simulink model "model"  (Simulink 7.4)
settings: Solver=ode45  StartTime=0.0  StopTime=15  MaxStep=2e-2  RelTol=1e-3
values from neighbouring files (symbols this model uses):
  Bm = 3e-6    (= 3e-06)    [beammodelparameters.m]    (also in project.mat)
  g = 9.8    [beammodelparameters.m]    (also in project.mat)
  Gv = 4    [beammodelparameters.m]    (also in project.mat)
  Jeff = Jm + Jg + Js    (= 5.66e-05)    [beammodelparameters.m]    (also in project.mat)
  K = (2/5)*(R/r)^2    (= 1.11111111111)    [beammodelparameters.m]    (also in project.mat)
  Ks = 10    [beammodelparameters.m]    (also in project.mat)
  Kt = 0.125    [beammodelparameters.m]    (also in project.mat = 0.225)
  Lm = 7.5e-3    (= 0.0075)    [beammodelparameters.m]    (also in project.mat = 0.025)
  M = 1 + (2/5)*(R/r)^2    (= 2.11111111111)    [beammodelparameters.m]    (also in lamdesign.m = p(nd+1:end).'; project.mat)
  N = 100    [beammodelparameters.m]    (also in lamdesign.m = [zeros(nd-nn,1);N]; project.mat)
  Rm = 4    [beammodelparameters.m]    (also in project.mat = 8)
  theta_o = 0.1    [beammodelparameters.m]    (also in project.mat)
  Vlim = 50    [beammodelparameters.m]    (also in project.mat)
  x_o = 0.25    [beammodelparameters.m]    (also in project.mat)
undefined symbols (not defined in the file or in its folder): Fn, Fp
settings Model: Creator=Duane  LastModifiedBy=Cam  ExtModeAutoUpdateStatusClock=off
settings DebuggingCC: SolverPrmCheckMsg=none

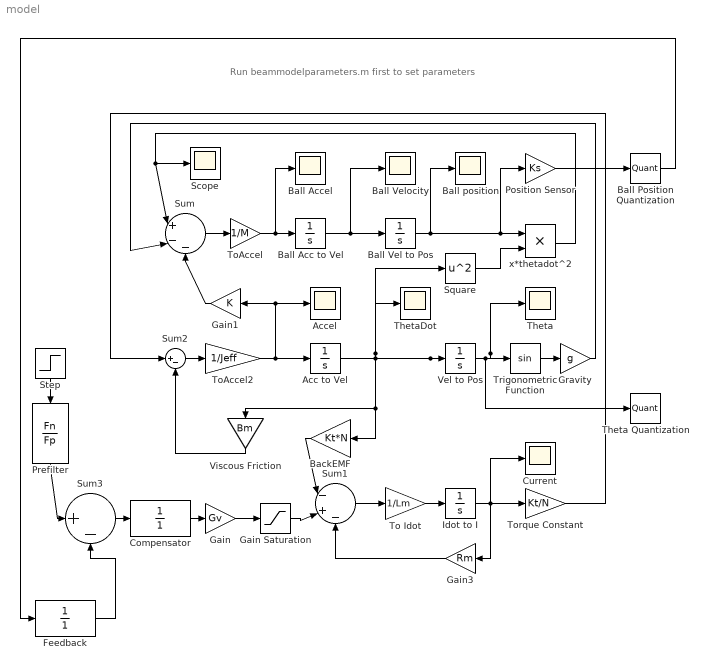
== system model ==
  note: Run beammodelparameters.m first to set parameters
  Acc to Vel : Integrator
  Accel : Scope
      settings: SaveName=ScopeData5
  BackEMF : Gain  Gain=Kt*N  ParameterDataType=fixdt(1, 16)  ParameterScaling=2^0  OutDataType=fixdt(1, 16)  OutScaling=2^0
  Ball Acc to Vel : Integrator
  Ball Accel : Scope
      settings: SaveName=ScopeData6
  Ball Position Quantization : Quantizer  QuantizationInterval=Xquant
  Ball Vel to Pos : Integrator  InitialCondition=x_o
  Ball Velocity : Scope
  Ball position : Scope
  Compensator : TransferFcn  Numerator=1  Denominator=1
  Current : Scope
      settings: SaveName=ScopeData4
  Feedback : TransferFcn  Numerator=1  Denominator=1
  Gain : Gain  Gain=Gv  ParameterDataType=fixdt(1, 16)  ParameterScaling=2^0  OutDataType=fixdt(1, 16)  OutScaling=2^0
  Gain Saturation : Saturate  UpperLimit=Vlim  LowerLimit=-Vlim  OutDataType=fixdt(1, 16)  OutScaling=2^0
  Gain1 : Gain  Gain=K  ParameterDataType=fixdt(1, 16)  ParameterScaling=2^0  OutDataType=fixdt(1, 16)  OutScaling=2^0
  Gain3 : Gain  Gain=Rm  ParameterDataType=fixdt(1, 16)  ParameterScaling=2^0  OutDataType=fixdt(1, 16)  OutScaling=2^0
  Gravity : Gain  Gain=g  ParameterDataType=fixdt(1, 16)  ParameterScaling=2^0  OutDataType=fixdt(1, 16)  OutScaling=2^0
  Idot to I : Integrator
  Position Sensor : Gain  Gain=Ks  ParameterDataType=fixdt(1, 16)  ParameterScaling=2^0  OutDataType=fixdt(1, 16)  OutScaling=2^0
  Prefilter : TransferFcn  Numerator=Fn  Denominator=Fp
  Scope : Scope
      settings: SaveName=ScopeData7
  Square : Math  Operator=square  OutDataType=fixdt(1, 16)  OutScaling=2^0  SaturateOnIntegerOverflow=on
  Step : Step  After=.05  SampleTime=0
  Sum : Sum  Inputs=|+--  OutDataType=fixdt(1, 16)  OutScaling=2^0
  Sum1 : Sum  Inputs=|-+-  OutDataType=fixdt(1, 16)  OutScaling=2^0
  Sum2 : Sum  Inputs=|+-  OutDataType=fixdt(1, 16)  OutScaling=2^0
  Sum3 : Sum  Inputs=|+-  OutDataType=fixdt(1, 16)  OutScaling=2^0
  Theta : Scope
      settings: SaveName=ScopeData2
  Theta Quantization : Quantizer  QuantizationInterval=Tquant
  ThetaDot : Scope
      settings: SaveName=ScopeData3
  To Idot : Gain  Gain=1/Lm  ParameterDataType=fixdt(1, 16)  ParameterScaling=2^0  OutDataType=fixdt(1, 16)  OutScaling=2^0
  ToAccel : Gain  Gain=1/M  ParameterDataType=fixdt(1, 16)  ParameterScaling=2^0  OutDataType=fixdt(1, 16)  OutScaling=2^0
  ToAccel2 : Gain  Gain=1/Jeff  ParameterDataType=fixdt(1, 16)  ParameterScaling=2^0  OutDataType=fixdt(1, 16)  OutScaling=2^0
  Torque Constant : Gain  Gain=Kt/N  ParameterDataType=fixdt(1, 16)  ParameterScaling=2^0  OutDataType=fixdt(1, 16)  OutScaling=2^0
  Trigonometric Function : Trigonometry
  Vel to Pos : Integrator  InitialCondition=theta_o
  Viscous Friction : Gain  Gain=Bm  ParameterDataType=fixdt(1, 16)  ParameterScaling=2^0  OutDataType=fixdt(1, 16)  OutScaling=2^0
  x*thetadot^2 : Product  Inputs=**  OutDataType=fixdt(1, 16)  OutScaling=2^-10
  wires:
  Ball Acc to Vel/1 -> Ball Vel to Pos/1, Ball Velocity/1
  Vel to Pos/1 -> Theta/1, Trigonometric Function/1, Theta Quantization/1
  ToAccel/1 -> Ball Acc to Vel/1, Ball Accel/1
  Sum/1 -> ToAccel/1
  Square/1 -> x*thetadot^2/2
  Ball Vel to Pos/1 -> Ball position/1, x*thetadot^2/1, Position Sensor/1
  x*thetadot^2/1 -> Sum/1, Scope/1
  Acc to Vel/1 -> Vel to Pos/1, Square/1, Viscous Friction/1, BackEMF/1, ThetaDot/1
  Gain3/1 -> Sum1/3
  Idot to I/1 -> Torque Constant/1, Gain3/1, Current/1
  To Idot/1 -> Idot to I/1
  Sum1/1 -> To Idot/1
  Trigonometric Function/1 -> Gravity/1
  Gravity/1 -> Sum/2
  Gain/1 -> Gain Saturation/1
  Gain Saturation/1 -> Sum1/2
  ToAccel2/1 -> Acc to Vel/1, Accel/1, Gain1/1
  Sum2/1 -> ToAccel2/1
  Viscous Friction/1 -> Sum2/2
  Position Sensor/1 -> Ball Position Quantization/1
  Torque Constant/1 -> Sum2/1
  Gain1/1 -> Sum/3
  BackEMF/1 -> Sum1/1
  Feedback/1 -> Sum3/2
  Prefilter/1 -> Sum3/1
  Compensator/1 -> Gain/1
  Sum3/1 -> Compensator/1
  Step/1 -> Prefilter/1
  Ball Position Quantization/1 -> Feedback/1
